simulink model "Longitudinal_Stability_Model_trade"  (R2013a)
settings: Solver=ode45  StartTime=0.0  StopTime=30  RelTol=1e-6
values from neighbouring files (symbols this model uses):
  K = 0    [Controller_Design.m]    (also in T17.m = -3; Trade1.m = 3)
undefined symbols (not defined in the file or in its folder): Step_CMD
settings Model: Creator=Willdog  LastModifiedBy=Willdog

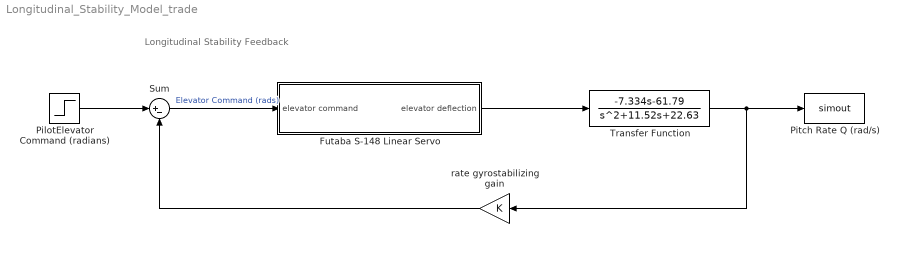
== system Longitudinal_Stability_Model_trade ==
  note: Longitudinal Stability Feedback
  Futaba S-148 Linear Servo : Subsystem  TreatAsAtomicUnit=on
  PilotElevator Command (radians) : Step  After=Step_CMD  SampleTime=0
  Pitch Rate Q (rad/s) : ToWorkspace  VariableName=simout  SampleTime=-1  SaveFormat=Timeseries
  Sum : Sum  Inputs=|+-
  Transfer Function : TransferFcn  Numerator=[-7.334 -61.79]  Denominator=[1 11.52 22.63]
  rate gyrostabilizing gain : Gain  Gain=K
  wires:
  rate gyrostabilizing gain/1 -> Sum/2
  Transfer Function/1 -> rate gyrostabilizing gain/1, Pitch Rate Q (rad/s)/1
  PilotElevator Command (radians)/1 -> Sum/1
  Sum/1 -> Futaba S-148 Linear Servo/1(elevator command)  "Elevator Command (rads)"
  Futaba S-148 Linear Servo/1(elevator deflection) -> Transfer Function/1

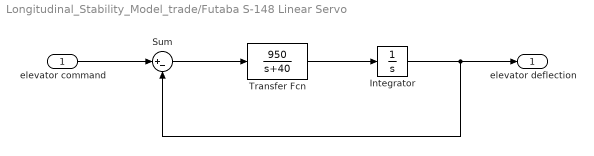
== system Longitudinal_Stability_Model_trade/Futaba S-148 Linear Servo ==
  elevator command : Inport
  Integrator : Integrator
  Sum : Sum  Inputs=|+-
  Transfer Fcn : TransferFcn  Numerator=[950]  Denominator=[1 40]
  elevator deflection : Outport
  wires:
  elevator command/1 -> Sum/1
  Sum/1 -> Transfer Fcn/1
  Transfer Fcn/1 -> Integrator/1
  Integrator/1 -> Sum/2, elevator deflection/1
